simulink model "Car_14DOF_Lat_Long_Control_BS_TEST"  (R2024b)
settings: Solver=ode4  StartTime=0.0  StopTime=60  FixedStep=0.001  RelTol=1e-3
undefined symbols (not defined in the file): c, C_line, curvature, gradbp, Iz, Kz1, Kz2, Kz3, lf, lh_vis, lr, psi0, Vx_test, x0, xRef2s, y0, yRef2s, z0
libraries: vehdynlibviscommon x1
settings Model: Creator=sherlock2204  LastModifiedBy=sherlock2204
settings DebuggingCC: SigSpecEnsureSampleTimeMsg=none

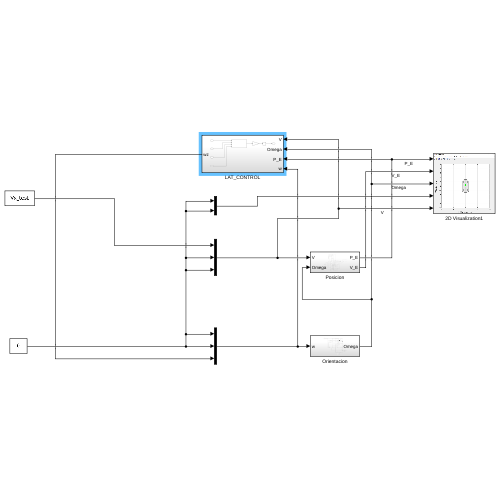
[thumbnail: Simulink's stored preview of the top-level diagram]
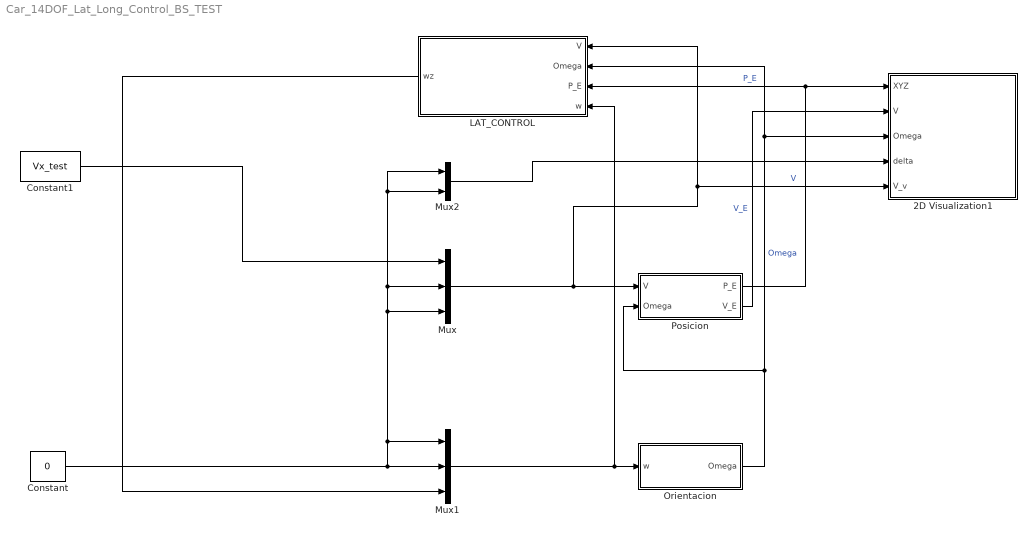
== system Car_14DOF_Lat_Long_Control_BS_TEST ==
  2D Visualization1 : Subsystem
      mask Display: image("visualization.JPG");
  Constant : Constant  Value=0
  Constant1 : Constant  Value=Vx_test
  LAT_CONTROL : Subsystem
  Mux : Mux  Inputs=3
  Mux1 : Mux  Inputs=3
  Mux2 : Mux  Inputs=2
  Orientacion : Subsystem
  Posicion : Subsystem
  wires:
  Mux/1 -> Posicion/1(V), LAT_CONTROL/1(V), 2D Visualization1/5(V_v)  "V"
  Orientacion/1(Omega) -> LAT_CONTROL/2(Omega), 2D Visualization1/3(Omega), Posicion/2(Omega)  "Omega"
  Posicion/2(V_E) -> 2D Visualization1/2(V)  "V_E"
  Posicion/1(P_E) -> 2D Visualization1/1(XYZ), LAT_CONTROL/3(P_E)  "P_E"
  Mux1/1 -> LAT_CONTROL/4(w), Orientacion/1(w)
  LAT_CONTROL/1(wz) -> Mux1/3
  Constant/1 -> Mux/2, Mux2/2, Mux2/1, Mux/3, Mux1/1, Mux1/2
  Constant1/1 -> Mux/1
  Mux2/1 -> 2D Visualization1/4(delta)

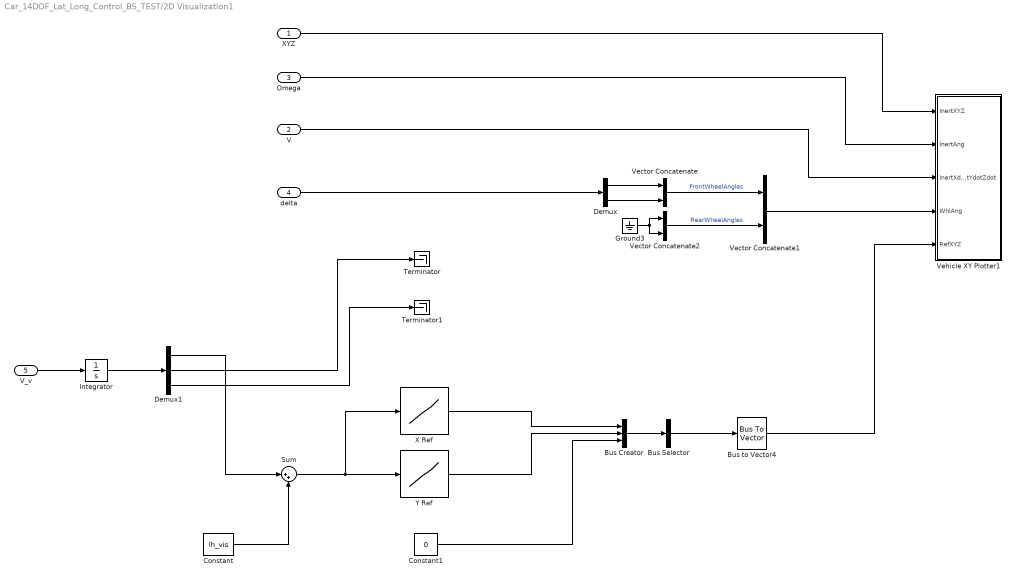
== system Car_14DOF_Lat_Long_Control_BS_TEST/2D Visualization1 ==
  XYZ : Inport
  V : Inport  Port=2
  Omega : Inport  Port=3
  delta : Inport  Port=4
  V_v : Inport  Port=5
  Bus Creator : BusCreator  Inputs=3
  Bus Selector : BusSelector  OutputSignals=signal1,signal2,signal3  OutputAsBus=on
  Bus to Vector4 : BusToVector
  Constant : Constant  Value=lh_vis
  Constant1 : Constant  Value=0
  Demux : Demux  Outputs=2
  Demux1 : Demux  Outputs=3
  Ground3 : Ground
  Integrator : Integrator
  Sum : Sum  Inputs=|++
  Terminator : Terminator
  Terminator1 : Terminator
  Vector Concatenate : Concatenate
  Vector Concatenate1 : Concatenate
  Vector Concatenate2 : Concatenate
  Vehicle XY Plotter1 : Subsystem  mask(Vehicle XY Plotter){extRef=on, extStats=off, extTireF=off, a=lf, b=lr, w=c, figBorder=10, bufferSize=1024, velNorm=5, tireFNorm=1000, pltDT=0.2}
      mask prompts: extRef "Plot path reference, extRef"; extStats "Display speed, RPM and Gear"; extTireF "Display tire forces"; a "Distance to front axle from CG, a [m]:"; b "Distance to rear axle from CG, b [m]:"; w "Track width, w [m]:"; figBorder "Distance to figure borders, figBorder [m]:"; bufferSize "Path buffer sampe size, bufferSize []:"; velNorm "Velocity vector scaling, velNorm [m*s/m]:"; tireFNorm "Tire force vector scaling, tireFNorm [m/N]:"; pltDT "Plot update rate, pltDT [s]:"
      mask help:
      | This block will display a MATLAB figure which indicates the vehicle path, current position and heading velocity.
      | An optional path reference is also provided.
      mask init:
      | block = gcb;
      | if autoblkschecksimstopped(block)
      |     ParamNames = {'extRef';'extStats';'extTireF';'extTireF'};
      |     PortNames = {'RefXYZ';'Stats';'TireFx';'TireFy'};
      |     for idx=1:length(PortNames)
      |         InportOption  = {'built-in/Ground', [PortNames{idx}, ' Ground'];...
      |             'built-in/Inport',PortNames{idx}};
      |         if ~strcmp(get_param(block,ParamNames{idx}),'on')
      |             NewBlkHdl = autoblksreplaceblock(block, InportOption, 1);
      |             set_param(NewBlkHdl, 'ShowName', 'off');
      |         else
      |             autoblksreplaceblock(block, InportOption, 2);
      |         end
      |     end
      |     InportNames = {'InertXYZ';'InertAng';'InertXdotYdotZdot';'WhlAng';'RefXYZ';'Stats';'TireFx';'TireFy'};
      |     FoundNames = get_param(find_system(block, 'LookUnderMasks', 'all', 'SearchDepth', 1, 'FollowLinks', 'on', 'BlockType', 'Inport'), 'Name');
      |     [~,PortI] = intersect(InportNames, FoundNames);
      |     PortI = sort(PortI);
      |     for idx = 1:length(PortI)
      |         set_param([block, '/', InportNames{PortI(idx)}], 'Port', num2str(idx));
      |     end
      | end
      mask TypeOptions a: Vehicle XY Plotter/a
      mask TypeOptions b: Vehicle XY Plotter/b
      mask TypeOptions w: Vehicle XY Plotter/w
      mask TypeOptions figBorder: Vehicle XY Plotter/figBorder
      mask TypeOptions bufferSize: Vehicle XY Plotter/bufferSize
      mask TypeOptions velNorm: Vehicle XY Plotter/velNorm
      mask TypeOptions tireFNorm: Vehicle XY Plotter/tireFNorm
      mask DialogControl Container3 Prompt: Plot and Display Options
  X Ref : Lookup_n-D  NumberOfTableDimensions=1  BreakpointsForDimension1=gradbp  Table=xRef2s  InternalRulePriority=Speed  RndMeth=Simplest
  Y Ref : Lookup_n-D  NumberOfTableDimensions=1  BreakpointsForDimension1=gradbp  Table=yRef2s  InternalRulePriority=Speed  RndMeth=Simplest
  wires:
  Omega/1 -> Vehicle XY Plotter1/2(InertAng)
  XYZ/1 -> Vehicle XY Plotter1/1(InertXYZ)
  V/1 -> Vehicle XY Plotter1/3(InertXdotYdotZdot)
  Vector Concatenate2/1 -> Vector Concatenate1/2  "RearWheelAngles"
  Vector Concatenate/1 -> Vector Concatenate1/1  "FrontWheelAngles"
  Ground3/1 -> Vector Concatenate2/2, Vector Concatenate2/1
  Vector Concatenate1/1 -> Vehicle XY Plotter1/4(WhlAng)
  delta/1 -> Demux/1
  Demux/1 -> Vector Concatenate/1
  Demux/2 -> Vector Concatenate/2
  Bus Creator/1 -> Bus Selector/1
  Y Ref/1 -> Bus Creator/2
  Bus Selector/1 -> Bus to Vector4/1
  Demux1/3 -> Terminator1/1
  X Ref/1 -> Bus Creator/1
  Constant1/1 -> Bus Creator/3
  Bus to Vector4/1 -> Vehicle XY Plotter1/5(RefXYZ)
  Demux1/2 -> Terminator/1
  V_v/1 -> Integrator/1
  Integrator/1 -> Demux1/1
  Demux1/1 -> Sum/1
  Sum/1 -> X Ref/1, Y Ref/1
  Constant/1 -> Sum/2

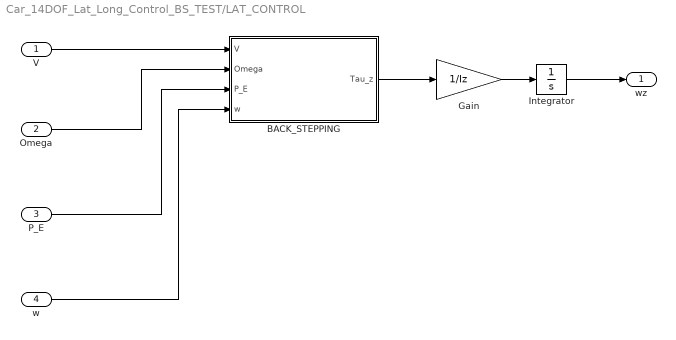
== system Car_14DOF_Lat_Long_Control_BS_TEST/LAT_CONTROL ==
  V : Inport
  Omega : Inport  Port=2
  P_E : Inport  Port=3
  w : Inport  Port=4
  BACK_STEPPING : Subsystem
  Gain : Gain  Gain=1/Iz
  Integrator : Integrator
  wz : Outport
  wires:
  V/1 -> BACK_STEPPING/1(V)
  Omega/1 -> BACK_STEPPING/2(Omega)
  P_E/1 -> BACK_STEPPING/3(P_E)
  w/1 -> BACK_STEPPING/4(w)
  BACK_STEPPING/1(Tau_z) -> Gain/1
  Gain/1 -> Integrator/1
  Integrator/1 -> wz/1

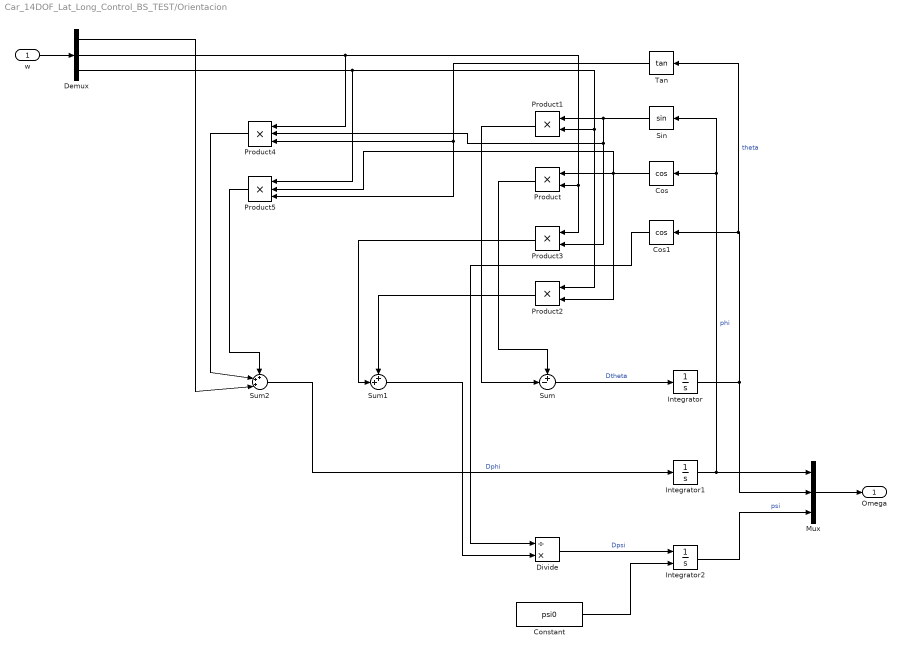
== system Car_14DOF_Lat_Long_Control_BS_TEST/Orientacion ==
  w : Inport
  Constant : Constant  Value=psi0
  Cos : Trigonometry  Operator=cos
  Cos1 : Trigonometry  Operator=cos
  Demux : Demux  Outputs=3
  Divide : Product  Inputs=/*
  Integrator : Integrator
  Integrator1 : Integrator
  Integrator2 : Integrator  InitialConditionSource=external
  Mux : Mux  Inputs=3
  Product{,1..3} (4 alike) : Product
  Product4 : Product  Inputs=3
  Product5 : Product  Inputs=3
  Sin : Trigonometry
  Sum : Sum  Inputs=+-|
  Sum1 : Sum  Inputs=++|
  Sum2 : Sum  Inputs=+++|
  Tan : Trigonometry  Operator=tan
  Omega : Outport
  wires:
  w/1 -> Demux/1
  Integrator/1 -> Mux/2, Tan/1, Cos1/1  "theta"
  Integrator2/1 -> Mux/3  "psi"
  Sin/1 -> Product4/2, Product3/2, Product1/1
  Cos/1 -> Product5/2, Product2/2, Product/1
  Demux/2 -> Product4/1, Product3/1, Product/2
  Demux/3 -> Product5/1, Product2/1, Product1/2
  Product/1 -> Sum/1
  Product1/1 -> Sum/2
  Sum/1 -> Integrator/1  "Dtheta"
  Integrator1/1 -> Sin/1, Cos/1, Mux/1  "phi"
  Product2/1 -> Sum1/1
  Product3/1 -> Sum1/2
  Divide/1 -> Integrator2/1  "Dpsi"
  Sum1/1 -> Divide/2
  Cos1/1 -> Divide/1
  Tan/1 -> Product4/3, Product5/3
  Sum2/1 -> Integrator1/1  "Dphi"
  Product5/1 -> Sum2/1
  Product4/1 -> Sum2/2
  Demux/1 -> Sum2/3
  Mux/1 -> Omega/1
  Constant/1 -> Integrator2/2

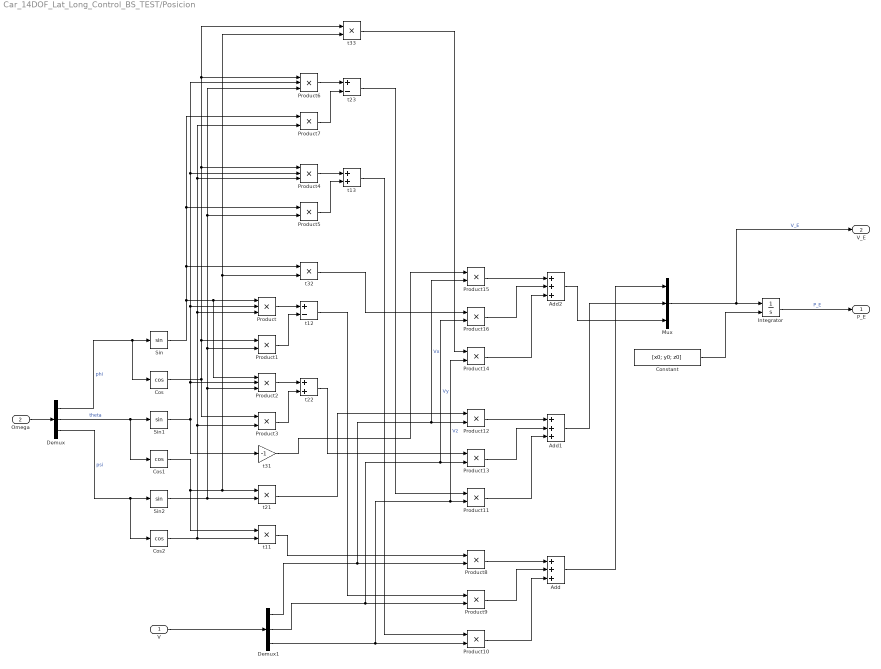
== system Car_14DOF_Lat_Long_Control_BS_TEST/Posicion ==
  V : Inport
  Omega : Inport  Port=2
  Add : Sum  Inputs=+++
  Add1 : Sum  Inputs=+++
  Add2 : Sum  Inputs=+++
  Constant : Constant  Value=[x0; y0; z0]
  Cos : Trigonometry  Operator=cos
  Cos1 : Trigonometry  Operator=cos
  Cos2 : Trigonometry  Operator=cos
  Demux : Demux  Outputs=3
  Demux1 : Demux  Outputs=3
  Integrator : Integrator  InitialConditionSource=external
  Mux : Mux  Inputs=3
  Product{,2,4,6} (4 alike) : Product  Inputs=3
  Product{1,3,5,7..16} (13 alike) : Product
  Sin : Trigonometry
  Sin1 : Trigonometry
  Sin2 : Trigonometry
  t{11,21,32..33} (4 alike) : Product
  t12 : Sum  Inputs=+-
  t13 : Sum
  t22 : Sum
  t23 : Sum  Inputs=+-
  t31 : Gain  Gain=-1
  P_E : Outport
  V_E : Outport  Port=2
  wires:
  Demux/1 -> Cos/1, Sin/1  "phi"
  Demux/2 -> Cos1/1, Sin1/1  "theta"
  Demux/3 -> Cos2/1, Sin2/1  "psi"
  Omega/1 -> Demux/1
  Cos2/1 -> Product7/2, Product4/3, Product/3, Product3/2, t11/2
  Cos1/1 -> t21/1, t33/2, t32/2, t11/1
  Sin2/1 -> Product6/3, Product5/2, Product1/2, Product2/3, t21/2
  Sin1/1 -> Product6/2, Product4/2, Product/2, Product2/2, t31/1
  Sin/1 -> Product7/1, Product5/1, t32/1, Product2/1, Product/1
  Cos/1 -> t33/1, Product6/1, Product4/1, Product1/1, Product3/1
  Product/1 -> t12/1
  Product1/1 -> t12/2
  Product3/1 -> t22/2
  Product2/1 -> t22/1
  Product5/1 -> t13/2
  Product4/1 -> t13/1
  Product6/1 -> t23/1
  Product7/1 -> t23/2
  V/1 -> Demux1/1
  Demux1/1 -> Product15/2, Product12/2, Product8/2  "Vx"
  Demux1/3 -> Product10/2, Product14/2, Product11/2  "Vz"
  Demux1/2 -> Product9/2, Product16/2, Product13/2  "Vy"
  t11/1 -> Product8/1
  t12/1 -> Product9/1
  t13/1 -> Product10/1
  Product8/1 -> Add/1
  Product9/1 -> Add/2
  Product10/1 -> Add/3
  Product13/1 -> Add1/2
  Product12/1 -> Add1/1
  Product11/1 -> Add1/3
  t21/1 -> Product12/1
  t22/1 -> Product13/1
  t23/1 -> Product11/1
  Product15/1 -> Add2/1
  Product16/1 -> Add2/2
  Product14/1 -> Add2/3
  t31/1 -> Product15/1
  t32/1 -> Product16/1
  t33/1 -> Product14/1
  Add/1 -> Mux/1
  Add1/1 -> Mux/2
  Add2/1 -> Mux/3
  Mux/1 -> V_E/1, Integrator/1  "V_E"
  Integrator/1 -> P_E/1  "P_E"
  Constant/1 -> Integrator/2

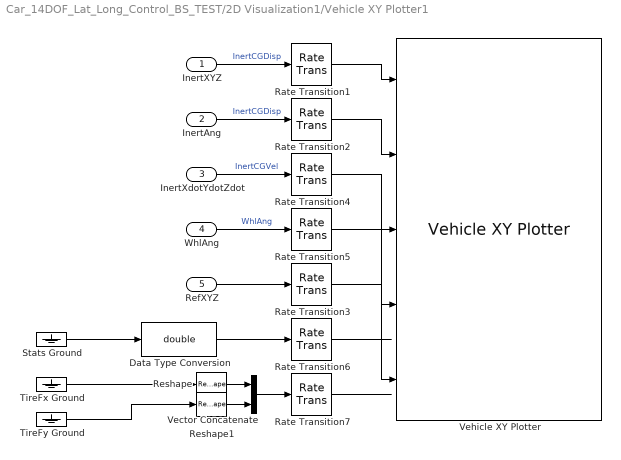
== system Car_14DOF_Lat_Long_Control_BS_TEST/2D Visualization1/Vehicle XY Plotter1 ==
  InertXYZ : Inport
  InertAng : Inport  Port=2
  InertXdotYdotZdot : Inport  Port=3
  WhlAng : Inport  Port=4
  RefXYZ : Inport  Port=5
  Data Type Conversion : DataTypeConversion  OutDataTypeStr=double  SaturateOnIntegerOverflow=off  RndMeth=Floor
  Rate Transition{1..7} (7 alike) : RateTransition  Deterministic=off  OutPortSampleTime=pltDT
  Reshape : Reshape  OutputDimensionality=Row vector (2-D)
  Reshape1 : Reshape  OutputDimensionality=Row vector (2-D)
  Stats Ground : Ground
  TireFx Ground : Ground
  TireFy Ground : Ground
  Vector Concatenate : Concatenate  Mode=Multidimensional array
  Vehicle XY Plotter : vehdynlibviscommon/Vehicle XY Plotter  w=w  a=a  b=b  figBorder=figBorder  bufferSize=bufferSize  extStats=off  extTireF=off
  wires:
  Stats Ground/1 -> Data Type Conversion/1
  InertAng/1 -> Rate Transition2/1  "InertCGDisp"
  InertXdotYdotZdot/1 -> Rate Transition4/1  "InertCGVel"
  InertXYZ/1 -> Rate Transition1/1  "InertCGDisp"
  WhlAng/1 -> Rate Transition5/1  "WhlAng"
  Rate Transition3/1 -> Vehicle XY Plotter/5
  Rate Transition1/1 -> Vehicle XY Plotter/1
  Rate Transition2/1 -> Vehicle XY Plotter/2
  Rate Transition4/1 -> Vehicle XY Plotter/3
  Rate Transition5/1 -> Vehicle XY Plotter/4
  Rate Transition6/1 -> ?
  Data Type Conversion/1 -> Rate Transition6/1
  Rate Transition7/1 -> ?
  Reshape/1 -> Vector Concatenate/1
  Reshape1/1 -> Vector Concatenate/2
  Vector Concatenate/1 -> Rate Transition7/1
  TireFx Ground/1 -> Reshape/1
  TireFy Ground/1 -> Reshape1/1
  RefXYZ/1 -> Rate Transition3/1

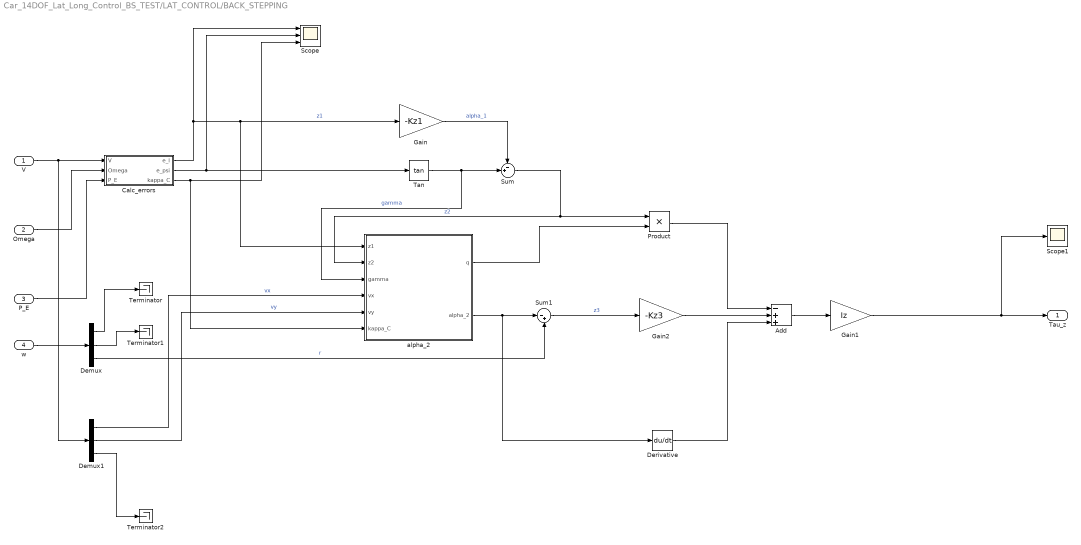
== system Car_14DOF_Lat_Long_Control_BS_TEST/LAT_CONTROL/BACK_STEPPING ==
  V : Inport
  Omega : Inport  Port=2
  P_E : Inport  Port=3
  w : Inport  Port=4
  Add : Sum  Inputs=-++
  Calc_errors : Subsystem
  Demux : Demux  Outputs=3
  Demux1 : Demux  Outputs=3
  Derivative : Derivative
  Gain : Gain  Gain=-Kz1
  Gain1 : Gain  Gain=Iz
  Gain2 : Gain  Gain=-Kz3
  Product : Product
  Scope : Scope  NumInputPorts=3
  Scope1 : Scope
  Sum : Sum  Inputs=-+|
  Sum1 : Sum  Inputs=|-+
  Tan : Trigonometry  Operator=tan
  Terminator : Terminator
  Terminator1 : Terminator
  Terminator2 : Terminator
  alpha_2 : Subsystem
  Tau_z : Outport
  wires:
  V/1 -> Calc_errors/1(V), Demux1/1
  Omega/1 -> Calc_errors/2(Omega)
  P_E/1 -> Calc_errors/3(P_E)
  Calc_errors/1(e_l) -> Scope/1, alpha_2/1(z1), Gain/1  "z1"
  Gain/1 -> Sum/1  "alpha_1"
  Tan/1 -> alpha_2/3(gamma), Sum/2  "gamma"
  w/1 -> Demux/1
  Demux/2 -> Terminator1/1
  Demux/1 -> Terminator/1
  Sum/1 -> Product/1, alpha_2/2(z2)  "z2"
  Demux1/3 -> Terminator2/1
  Demux1/1 -> alpha_2/4(vx)  "vx"
  Demux1/2 -> alpha_2/5(vy)  "vy"
  Calc_errors/3(kappa_C) -> Scope/3, alpha_2/6(kappa_C)
  alpha_2/2(alpha_2) -> Sum1/1, Derivative/1
  Demux/3 -> Sum1/2  "r"
  Sum1/1 -> Gain2/1  "z3"
  alpha_2/1(q) -> Product/2
  Gain2/1 -> Add/2
  Derivative/1 -> Add/3
  Product/1 -> Add/1
  Add/1 -> Gain1/1
  Gain1/1 -> Scope1/1, Tau_z/1
  Calc_errors/2(e_psi) -> Scope/2, Tan/1

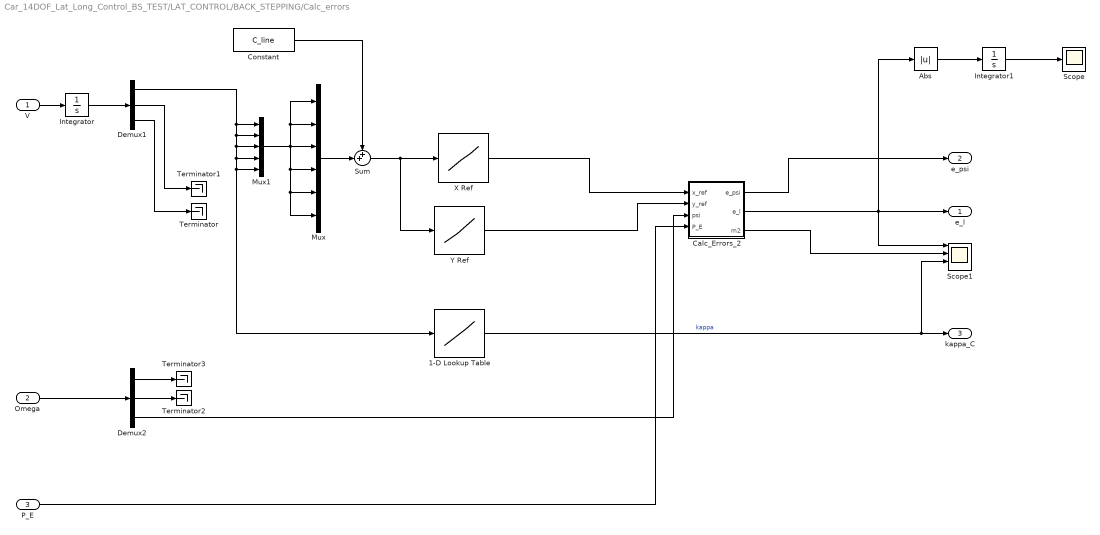
== system Car_14DOF_Lat_Long_Control_BS_TEST/LAT_CONTROL/BACK_STEPPING/Calc_errors ==
  V : Inport
  Omega : Inport  Port=2
  P_E : Inport  Port=3
  1-D Lookup Table : Lookup_n-D  NumberOfTableDimensions=1  BreakpointsForDimension1=gradbp  Table=curvature  InternalRulePriority=Speed  RndMeth=Simplest
  Abs : Abs  SaturateOnIntegerOverflow=off
  Calc_Errors_2 : MATLAB Function  TreatAsAtomicUnit=on
  Constant : Constant  Value=C_line
  Demux1 : Demux  Outputs=3
  Demux2 : Demux  Outputs=3
  Integrator : Integrator
  Integrator1 : Integrator
  Mux : Mux  Inputs=6
  Mux1 : Mux  Inputs=5
  Scope : Scope
  Scope1 : Scope  NumInputPorts=4
  Sum : Sum  Inputs=++|
  Terminator{,1..3} (4 alike) : Terminator
  X Ref : Lookup_n-D  NumberOfTableDimensions=1  BreakpointsForDimension1=gradbp  Table=xRef2s  InternalRulePriority=Speed  RndMeth=Simplest
  Y Ref : Lookup_n-D  NumberOfTableDimensions=1  BreakpointsForDimension1=gradbp  Table=yRef2s  InternalRulePriority=Speed  RndMeth=Simplest
  e_l : Outport
  e_psi : Outport  Port=2
  kappa_C : Outport  Port=3
  wires:
  Mux/1 -> Sum/2
  Sum/1 -> X Ref/1, Y Ref/1
  V/1 -> Integrator/1
  Demux1/1 -> 1-D Lookup Table/1, Mux1/5, Mux1/4, Mux1/3, Mux1/2, Mux1/1
  Integrator/1 -> Demux1/1
  Demux1/3 -> Terminator/1
  Constant/1 -> Sum/1
  X Ref/1 -> Calc_Errors_2/1(x_ref)
  Demux2/1 -> Terminator3/1
  Demux2/2 -> Terminator2/1
  Demux1/2 -> Terminator1/1
  Y Ref/1 -> Calc_Errors_2/2(y_ref)
  Omega/1 -> Demux2/1
  Demux2/3 -> Calc_Errors_2/3(psi)
  P_E/1 -> Calc_Errors_2/4(P_E)
  1-D Lookup Table/1 -> Scope1/3, kappa_C/1  "kappa"
  Mux1/1 -> Mux/6, Mux/5, Mux/4, Mux/3, Mux/1, Mux/2
  Calc_Errors_2/1(e_psi) -> e_psi/1
  Calc_Errors_2/2(e_l) -> Abs/1, e_l/1, Scope1/1
  Calc_Errors_2/3(m2) -> Scope1/2
  Integrator1/1 -> Scope/1
  Abs/1 -> Integrator1/1

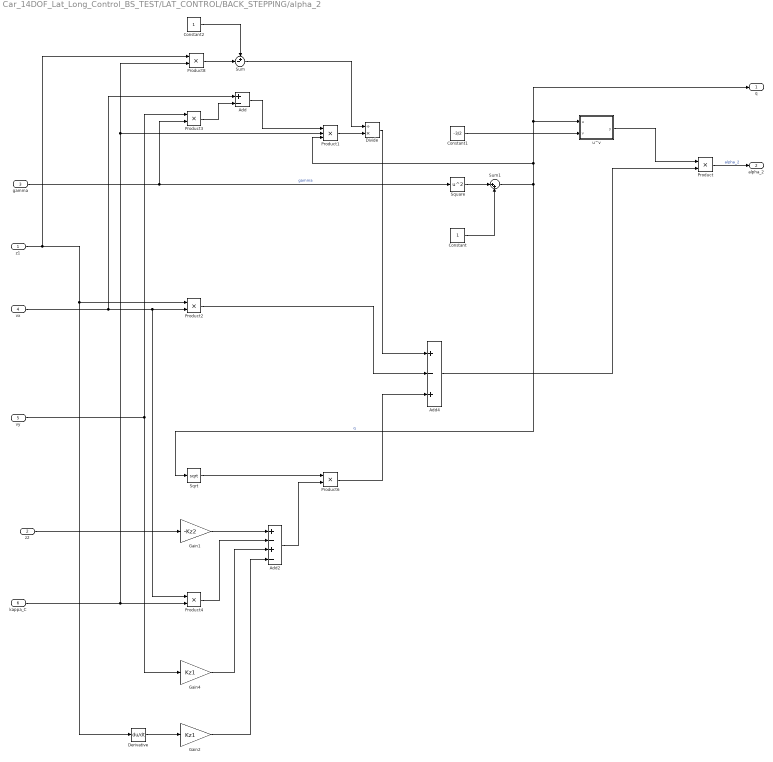
== system Car_14DOF_Lat_Long_Control_BS_TEST/LAT_CONTROL/BACK_STEPPING/alpha_2 ==
  z1 : Inport
  z2 : Inport  Port=2
  gamma : Inport  Port=3
  vx : Inport  Port=4
  vy : Inport  Port=5
  kappa_C : Inport  Port=6
  Add : Sum  Inputs=+-
  Add2 : Sum  Inputs=+-+-
  Add4 : Sum  Inputs=+-+
  Constant : Constant
  Constant1 : Constant  Value=-3/2
  Constant2 : Constant
  Derivative : Derivative
  Divide : Product  Inputs=/*
  Gain1 : Gain  Gain=-Kz2
  Gain2 : Gain  Gain=Kz1
  Gain4 : Gain  Gain=Kz1
  Product{,2..4,6,8} (6 alike) : Product
  Product1 : Product  Inputs=3
  Sqrt : Sqrt
  Square : Math  Operator=square
  Sum : Sum  Inputs=+-|
  Sum1 : Sum  Inputs=|++
  u^v : MATLAB Function  TreatAsAtomicUnit=on
  q : Outport
  alpha_2 : Outport  Port=2
  wires:
  Sqrt/1 -> Product6/1
  Constant/1 -> Sum1/2
  Square/1 -> Sum1/1
  gamma/1 -> Product3/2, Square/1  "gamma"
  Sum1/1 -> Sqrt/1, u^v/1(u), q/1, Product1/3  "q"
  u^v/1(y) -> Product/1
  Constant1/1 -> u^v/2(v)
  vx/1 -> Add/1, Product4/1, Product2/2
  z1/1 -> Product8/1, Derivative/1, Product2/1
  vy/1 -> Product3/1, Gain4/1
  z2/1 -> Gain1/1
  kappa_C/1 -> Product1/2, Product8/2, Product4/2
  Gain1/1 -> Add2/1
  Product4/1 -> Add2/2
  Gain4/1 -> Add2/3
  Add2/1 -> Product6/2
  Product6/1 -> Add4/3
  Product2/1 -> Add4/2
  Add/1 -> Product1/1
  Product3/1 -> Add/2
  Product1/1 -> Divide/2
  Constant2/1 -> Sum/1
  Sum/1 -> Divide/1
  Product8/1 -> Sum/2
  Divide/1 -> Add4/1
  Add4/1 -> Product/2
  Product/1 -> alpha_2/1  "alpha_2"
  Derivative/1 -> Gain2/1
  Gain2/1 -> Add2/4

== matlab function Car_14DOF_Lat_Long_Control_BS_TEST/LAT_CONTROL/BACK_STEPPING/Calc_errors/Calc_Errors_2 ==
  data: x_ref input; e_psi output; y_ref input; psi input; P_E input; e_l output; m2 output
function [e_psi, e_l,m2] = fcn(x_ref,y_ref,psi,P_E)

P = polyfit(x_ref,y_ref,1);
m2 = P(1);
b2 = P(2);
x1 = 0;
y1 = b2;
x2 = 1;
y2 = m2*x2+b2;
psi_ref = atan2(y2-y1,x2-x1);
%psi_ref = atan(m);
e_psi = psi-psi_ref;

% Traslacion al lugar donde esta el punto S
x_s = P_E(1)-x_ref(16);
y_s = P_E(2)-y_ref(16);
% Rotacion a la misma orientacion del coche
y_c = x_s*sin(-psi_ref)+y_s*cos(-psi_ref);
e_l = y_c;

== matlab function Car_14DOF_Lat_Long_Control_BS_TEST/LAT_CONTROL/BACK_STEPPING/alpha_2/u^v ==
  data: u input; y output; v input
function y = fcn(u,v)

y = u^(v);
